simulink model "SimulTaller"  (R2020b)
settings: Solver=VariableStepAuto  StartTime=0.0  StopTime=10  RelTol=1e-3
values from neighbouring files (symbols this model uses):
  h = 0.1    [Taller2.m]
  L = dlqr(Ae,Be,Q,R)    [Taller2.m]
  X0 = [10; -pi/4; 0; 0]    [Taller2.m]
undefined symbols (not defined in the file or in its folder): Az, Bz
settings Model: Creator=Eduard  LastModifiedBy=Eduard

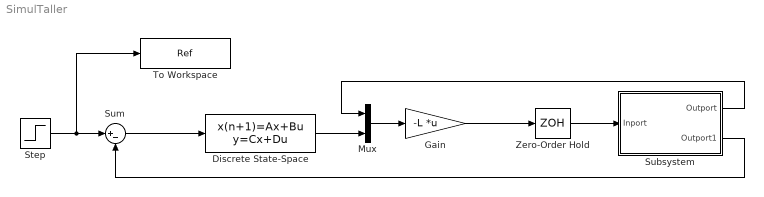
== system SimulTaller ==
  Discrete State-Space : DiscreteStateSpace  A=Az  B=Bz  C=eye(size(Az))  D=zeros(size(Bz))  SampleTime=h
  Gain : Gain  Gain=-L  Multiplication=Matrix(K*u) (u vector)
  Mux : Mux  Inputs=2
  Step : Step  Time=0  After=10  SampleTime=h
  Subsystem : Subsystem
  Sum : Sum  Inputs=|+-
  To Workspace : ToWorkspace  VariableName=Ref  SaveFormat=Structure With Time  SampleTime=h
  Zero-Order Hold : ZeroOrderHold  SampleTime=h
  wires:
  Step/1 -> To Workspace/1, Sum/1
  Sum/1 -> Discrete State-Space/1
  Discrete State-Space/1 -> Mux/2
  Mux/1 -> Gain/1
  Gain/1 -> Zero-Order Hold/1
  Zero-Order Hold/1 -> Subsystem/1(Inport)
  Subsystem/1(Outport) -> Mux/1
  Subsystem/2(Outport1) -> Sum/2

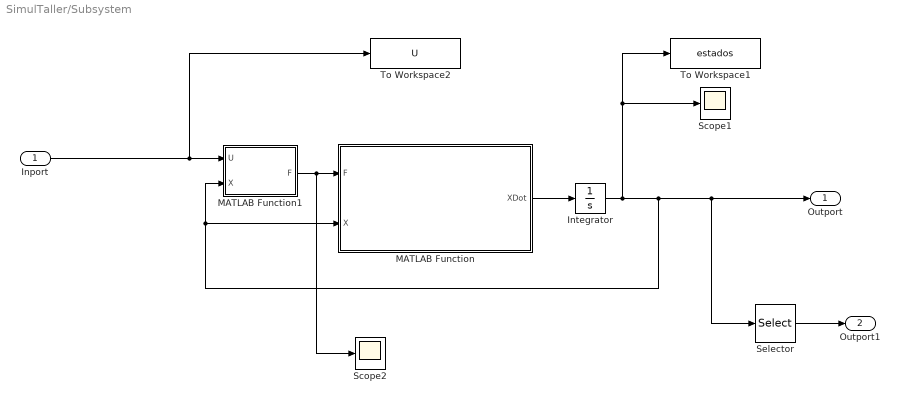
== system SimulTaller/Subsystem ==
  Inport : Inport
  Integrator : Integrator  InitialCondition=X0
  MATLAB Function : MATLAB Function  TreatAsAtomicUnit=on
  MATLAB Function1 : MATLAB Function  TreatAsAtomicUnit=on
  Scope1 : Scope
  Scope2 : Scope
  Selector : Selector  InputPortWidth=4  IndexOptions=Index vector (dialog)  Indices=2  OutputSizes=1
  To Workspace1 : ToWorkspace  VariableName=estados  SaveFormat=Structure With Time  SampleTime=h
  To Workspace2 : ToWorkspace  VariableName=U  SaveFormat=Structure With Time  SampleTime=h
  Outport : Outport
  Outport1 : Outport  Port=2
  wires:
  MATLAB Function/1(XDot) -> Integrator/1
  Inport/1 -> To Workspace2/1, MATLAB Function1/1(U)
  Integrator/1 -> To Workspace1/1, Scope1/1, Selector/1, Outport/1, MATLAB Function/2(X), MATLAB Function1/2(X)
  Selector/1 -> Outport1/1
  MATLAB Function1/1(F) -> Scope2/1, MATLAB Function/1(F)

== matlab function SimulTaller/Subsystem/MATLAB Function1 ==
  data: U input; F output; X input
function F = fcn(U,X)
[m,J,r,g]           = deal(10,0.1,0.5,9.8);

f1 = (m*r*U(1)+J*cos(X(2))*U(2)+m*g*r)/(2*cos(X(2))*r);
f2 = (m*r*U(1)-J*cos(X(2))*U(2)+m*g*r)/(2*cos(X(2))*r);
F = [f1;f2];
end

== matlab function SimulTaller/Subsystem/MATLAB Function ==
  data: F input; XDot output; X input
function XDot  = modelo_nolineal(F,X)
% Constantes del modelo
[m,J,r,g]           = deal(10,0.1,0.5,9.8);
% Estados
[X1,X2,X3,X4]= deal(X(1),X(2),X(3),X(4));
% Derivadas de los estados
x1p = X3;
x2p = X4;
x3p = -g + (1/m)*cos(X2)*(F(1) + F(2));
x4p = (r/J)*(F(1)- F(2));
%% Modelo en espacio de estados
XDot                = [x1p; x2p; x3p; x4p];
end
